simulink model "PIDdmasf"  (R2016a)
settings: Solver=FixedStepDiscrete  StartTime=0.0  StopTime=20
libraries: simulink x2, fuzblock x1
settings Model: Creator=PC  LastModifiedBy=PC
settings SolverCC: MaxConsecutiveZCs=10000  SolverJacobianMethodControl=FullAnalytical  ZeroCrossControl=DisableAll  ZeroCrossAlgorithm=Adaptive  AutoInsertRateTranBlk=on
settings DataIOCC: LimitDataPoints=on  SaveOutput=off  SaveTime=off  Refine=10
settings OptimizationCC: ExpressionDepthLimit=2147483647  LifeSpan=1
settings DebuggingCC: UnderspecifiedInitializationDetection=Classic  MergeDetectMultiDrivingBlocksExec=none  FcnCallInpInsideContextMsg=EnableAllAsWarning  AllowSymbolicDim=off  StateNameClashWarn=warning
settings GRTTargetCC: CombineOutputUpdateFcns=off  GRTInterface=on

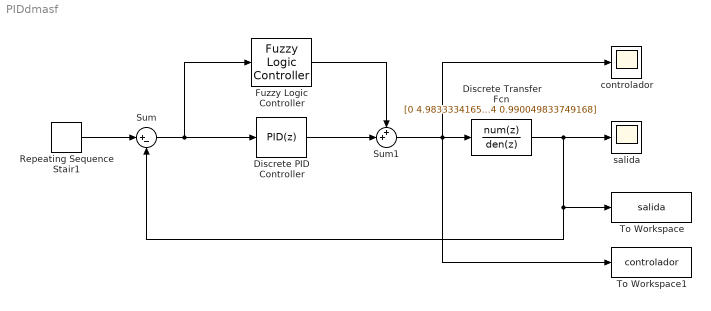
== system PIDdmasf ==
  Discrete Transfer Fcn : DiscreteTransferFcn  Numerator=[0 4.98333341652778e-05 4.96674991666667e-05]  Denominator=[1 -1.98995033291584 0.990049833749168]  SampleTime=0.01
  Discrete PID Controller : simulink/Continuous/PID Controller  Controller=PID  TimeDomain=Discrete-time  SampleTime=0.01  IntegratorMethod=Trapezoidal  FilterMethod=Backward Euler  Form=Parallel  UseFilter=off  ControllerParametersSource=internal  P=0.2  I=1  D=1  N=100  InitialConditionSource=internal  InitialConditionForIntegrator=0  InitialConditionForFilter=0  ExternalReset=none  LimitOutput=off  UpperSaturationLimit=inf  LowerSaturationLimit=-inf  LinearizeAsGain=off  AntiWindupMode=none  Kb=1  TrackingMode=off  Kt=1  PParamMin=[]  PParamMax=[]  IParamMin=[]  IParamMax=[]  DParamMin=[]  DParamMax=[]  NParamMin=[]  NParamMax=[]  KbParamMin=[]  KbParamMax=[]  KtParamMin=[]  KtParamMax=[]  POutMin=[]  POutMax=[]  IOutMin=[]  IOutMax=[]  DOutMin=[]  DOutMax=[]  NOutMin=[]  NOutMax=[]  KbOutMin=[]  KbOutMax=[]  KtOutMin=[]  KtOutMax=[]  IntegratorOutMin=[]  IntegratorOutMax=[]  FilterOutMin=[]  FilterOutMax=[]  SumOutMin=[]  SumOutMax=[]  SumI1OutMin=[]  SumI1OutMax=[]  SumI2OutMin=[]  SumI2OutMax=[]  SumI3OutMin=[]  SumI3OutMax=[]  SumDOutMin=[]  SumDOutMax=[]  SaturationOutMin=[]  SaturationOutMax=[]  IntegratorContinuousStateAttributes=''  IntegratorStateMustResolveToSignalObject=off  IntegratorRTWStateStorageClass=Auto  FilterContinuousStateAttributes=''  FilterStateMustResolveToSignalObject=off  FilterRTWStateStorageClass=Auto  DifferentiatorICPrevScaledInput=0  DifferentiatorOutMin=[]  DifferentiatorOutMax=[]
  Fuzzy Logic Controller : fuzblock/Fuzzy Logic  Controller  fis='simpleF.fis'
  Repeating Sequence Stair1 : simulink/Sources/Repeating Sequence Stair  OutValues=[1 1].'  tsamp=0.01  OutMin=[]  OutMax=[]  OutDataTypeStr=double  OutputDataTypeScalingMode=double  OutDataType=fixdt(0,8)  ConRadixGroup=Best Precision: Vector-wise  OutScaling=2^-12
  Sum : Sum  Inputs=|+-
  Sum1 : Sum  Inputs=++|
  To Workspace : ToWorkspace  VariableName=salida  SaveFormat=Timeseries  SampleTime=-1
  To Workspace1 : ToWorkspace  VariableName=controlador  SaveFormat=Timeseries  SampleTime=-1
  controlador : Scope
  "salida " : Scope
  wires:
  Discrete Transfer Fcn/1 -> "salida "/1, To Workspace/1, Sum/2
  Sum/1 -> Fuzzy Logic Controller/1, Discrete PID Controller/1
  Discrete PID Controller/1 -> Sum1/2
  Repeating Sequence Stair1/1 -> Sum/1
  Sum1/1 -> Discrete Transfer Fcn/1, To Workspace1/1, controlador/1
  Fuzzy Logic Controller/1 -> Sum1/1
